simulink model "lqg_test"  (R2015b)
settings: Solver=VariableStepAuto  StartTime=0.0  StopTime=80.0  RelTol=1e-3
values from neighbouring files (symbols this model uses):
  G1 = series(au,Gu)    [LQG_LTR.m]
undefined symbols (not defined in the file or in its folder): Ks_lqg, pulsazione
settings Model: Creator=michele  LastModifiedBy=michele

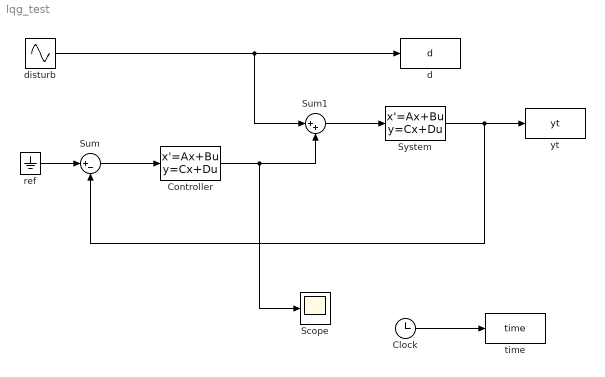
== system lqg_test ==
  Clock : Clock
  Controller : StateSpace  A=Ks_lqg.a  B=Ks_lqg.b  C=Ks_lqg.c  D=Ks_lqg.d  X0=0
  Scope : Scope
  Sum : Sum  Inputs=|+-
  Sum1 : Sum  Inputs=|++
  System : StateSpace  A=G1.NominalValue.a  B=G1.NominalValue.b  C=G1.NominalValue.c  D=G1.NominalValue.d  X0=0
  d : ToWorkspace  VariableName=d  SaveFormat=Timeseries  SampleTime=-1
  disturb : Sin  Frequency=pulsazione  SampleTime=0
  ref : Ground
  time : ToWorkspace  VariableName=time  SaveFormat=Timeseries  SampleTime=-1
  yt : ToWorkspace  VariableName=yt  SaveFormat=Timeseries  SampleTime=-1
  wires:
  Sum1/1 -> System/1
  System/1 -> Sum/2, yt/1
  Sum/1 -> Controller/1
  ref/1 -> Sum/1
  disturb/1 -> Sum1/1, d/1
  Clock/1 -> time/1
  Controller/1 -> Scope/1, Sum1/2
